simulink model "UnitDelayBio1MDLRef"  (R2017b)
settings: Solver=FixedStepDiscrete  StartTime=0.0  StopTime=19.8  FixedStep=0.200000  RelTol=1e-3  EnableMultiTasking=on
PreLoadFcn:
  | cellInfo =  {
  |   { ...
  |     'acs_command_msg', ...
  |     '', ...
  |     sprintf(''), { ...
  |       {'torque_com_wheel', 3, 'double', -1, 'real', 'Sample'}; ...
  |       {'thruster_on_times', 6, 'double', -1, 'real', 'Sample'}; ...
  |    }
  |   }
  | };
  | Simulink.Bus.cellToObject(cellInfo);
  | 
  | 
  | cellInfo = {
  |     { ...
  |          'command_state_msg' , ...
  |          '', ...
  |          sprintf(''), {  ...
  |                {  'q_com', 4, 'single', -1, 'real', 'Sample' }; ...
  |                {  'sm_spin_axis', 3, 'single', -1, 'real', 'Sample' }; ...
  |                {  'sm_rate_vec', 3, 'single', -1, 'real', 'Sample' }; ...
  |                {  'man_wheel_speed', 3, 'single', -1, 'real', 'Sample' }; ...
  |                {  'man_wheel_torq', 3, 'single', -1, 'real', 'Sample' }; ...
  |                {  'man_gimbal_cmd', 1, 'int16', -1, 'real', 'Sample' }; ...
  |                {  'man_prop_cmd', 8, 'uint16', -1, 'real', 'Sample' }; ...
  |                {  'gyro_LPF_on', 1, 'uint8', -1, 'real', 'Sample' }; ...
  |                {  'st_status', 1, 'uint8', -1, 'real', 'Sample' }; ...
  |                {  'mode', 1, 'uint8', -1, 'real', 'Sample' }; ...
  |                {  'KF_enable', 1, 'uint8', -1, 'real', 'Sample' }; ...
  |                {  'bypass_acs', 3, 'uint8', -1, 'real', 'Sample' }; ...
  |                {  'mm_flag', 1, 'uint8', -1, 'real', 'Sample' }; ...
  |          }
  |     }
  | };
  | Simulink.Bus.cellToObject(cellInfo);
  | 
  | dt = 0.2;
model workspace (MAT data in the model file):
  already_pp = 0
settings Model: Creator=hbourbou  LastModifiedBy=hbourbou
settings DataIOCC: LimitDataPoints=on  SaveFormat=Structure
settings OptimizationCC: LifeSpan=inf
settings DebuggingCC: AlgebraicLoopMsg=error  ArtificialAlgebraicLoopMsg=error  SFUnexpectedBacktrackingDiag=warning  SFNoUnconditionalDefaultTransitionDiag=warning  SFExecutionAtInitializationDiag=none
settings HardwareCC: ProdBitPerPointer=32  ProdBitPerSizeT=32  ProdBitPerPtrDiffT=32  ProdLargestAtomicFloat=None  ProdIntDivRoundTo=Undefined  ProdEndianess=Unspecified  ProdWordSize=32  ProdHWDeviceType=32-bit Generic
settings ModelReferenceCC: PropagateSignalLabelsOutOfModel=off
settings CodeAppCC: StateflowObjectComments=on
settings GRTTargetCC: TargetLangStandard=C89/C90 (ANSI)  GeneratePreprocessorConditionals=Disable all
settings ConfigComp: CovMetricSettings=dw  CovHtmlReporting=on  CovSaveCumulativeToWorkspaceVar=on  CovSaveSingleToWorkspaceVar=on  CovExternalEMLEnable=off

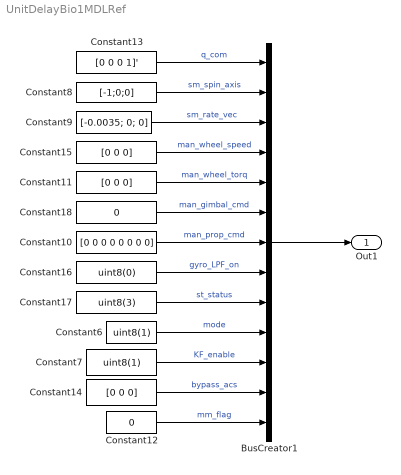
== system UnitDelayBio1MDLRef ==
  BusCreator1 : BusCreator  Inputs=13  OutDataTypeStr=Bus: command_state_msg  NonVirtualBus=on
      settings: InheritFromInputs=off
  Constant10 : Constant  Value=[0 0 0 0 0 0 0 0]  OutDataTypeStr=uint16  SampleTime=dt
  Constant11 : Constant  Value=[0 0 0]  OutDataTypeStr=single  SampleTime=dt
  Constant12 : Constant  Value=0  OutDataTypeStr=uint8  SampleTime=dt
  Constant13 : Constant  Value=[0 0 0 1]'  OutDataTypeStr=Inherit: Inherit via back propagation  SampleTime=dt
  Constant14 : Constant  Value=[0 0 0]  OutDataTypeStr=uint8  SampleTime=dt
  Constant15 : Constant  Value=[0 0 0]  OutDataTypeStr=single  SampleTime=dt
  Constant16 : Constant  Value=uint8(0)  SampleTime=dt
  Constant17 : Constant  Value=uint8(3)  SampleTime=dt
  Constant18 : Constant  Value=0  OutDataTypeStr=int16  SampleTime=dt
  Constant6 : Constant  Value=uint8(1)  SampleTime=dt
  Constant7 : Constant  Value=uint8(1)  SampleTime=dt
  Constant8 : Constant  Value=[-1;0;0]  OutDataTypeStr=Inherit: Inherit via back propagation  SampleTime=dt
  Constant9 : Constant  Value=[-0.0035; 0; 0]  OutDataTypeStr=Inherit: Inherit via back propagation  SampleTime=dt
  Out1 : Outport  OutDataTypeStr=Bus: command_state_msg
  wires:
  Constant18/1 -> BusCreator1/6  "man_gimbal_cmd"
  Constant9/1 -> BusCreator1/3  "sm_rate_vec"
  Constant7/1 -> BusCreator1/11  "KF_enable"
  Constant17/1 -> BusCreator1/9  "st_status"
  Constant10/1 -> BusCreator1/7  "man_prop_cmd"
  Constant14/1 -> BusCreator1/12  "bypass_acs"
  Constant11/1 -> BusCreator1/5  "man_wheel_torq"
  Constant15/1 -> BusCreator1/4  "man_wheel_speed"
  Constant12/1 -> BusCreator1/13  "mm_flag"
  Constant8/1 -> BusCreator1/2  "sm_spin_axis"
  Constant6/1 -> BusCreator1/10  "mode"
  Constant16/1 -> BusCreator1/8  "gyro_LPF_on"
  Constant13/1 -> BusCreator1/1  "q_com"
  BusCreator1/1 -> Out1/1
